simulink model "PasaBajo"  (R2020a)
settings: Solver=FixedStepAuto  StartTime=0.0  StopTime=6  FixedStep=0.003  RelTol=1e-3
undefined symbols (not defined in the file): wc
libraries: androidsensorlib x1
settings Model: Creator=luisi  LastModifiedBy=luisi
settings OptimizationCC: EnhancedBackFolding=on  PassReuseOutputArgsAs=Individual arguments  ZeroExternalMemoryAtStartup=off  ZeroInternalMemoryAtStartup=off  MaxStackSize=64  OptimizeBlockOrder=speed  DifferentSizesBufferReuse=on  EfficientTunableParamExpr=on
settings DebuggingCC: ParameterTunabilityLossMsg=error
settings HardwareCC: ProdBitPerPointer=32  ProdBitPerSizeT=32  ProdBitPerPtrDiffT=32  ProdLargestAtomicInteger=Long  ProdLargestAtomicFloat=Double  ProdWordSize=32  ProdHWDeviceType=ARM Compatible->ARM Cortex
settings SFSimCC: MATLABDynamicMemAlloc=off
settings RTWCC: SystemTargetFile=ert.tlc  HardwareBoard=Android Device  TemplateMakefile=ert_default_tmf  RTWVerbose=off  Toolchain=Android SDK/NDK Tools
settings CodeAppCC: ForceParamTrailComments=on  IgnoreCustomStorageClasses=off  OperatorAnnotations=on  SimulinkDataObjDesc=on  SFDataObjDesc=on  InsertBlockDesc=on
settings ERTTargetCC: SupportContinuousTime=on

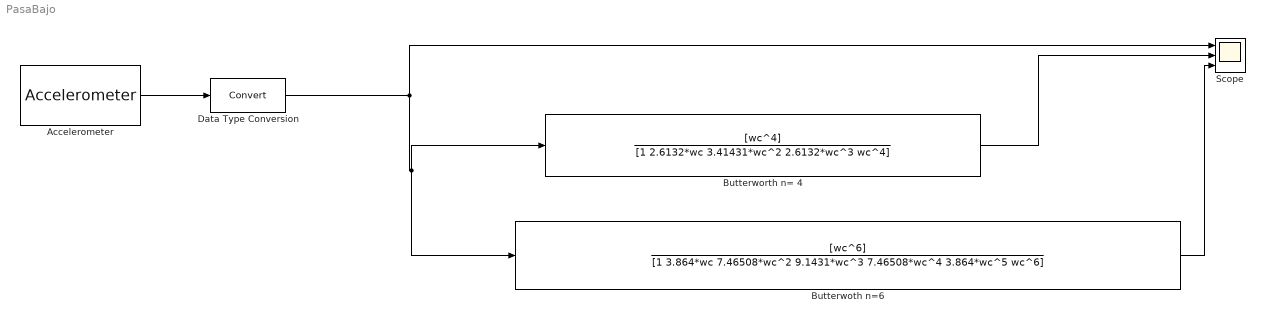
== system PasaBajo ==
  Accelerometer : androidsensorlib/Accelerometer  OutputVector=off  SampleTime=0.003  BlockPlatform=Android
      settings: SourceProductBaseCode=ANDROID
  Butterworth n= 4 : TransferFcn  Numerator=[wc^4]  Denominator=[1 2.6132*wc 3.41431*wc^2 2.6132*wc^3 wc^4]
  Butterwoth n=6 : TransferFcn  Numerator=[wc^6]  Denominator=[1 3.864*wc 7.46508*wc^2 9.1431*wc^3 7.46508*wc^4 3.864*wc^5 wc^6]
  Data Type Conversion : DataTypeConversion
  Scope : Scope  NumInputPorts=3
  wires:
  Data Type Conversion/1 -> Butterwoth n=6/1, Butterworth n= 4/1, Scope/1
  Accelerometer/2 -> Data Type Conversion/1
  Butterworth n= 4/1 -> Scope/2
  Butterwoth n=6/1 -> Scope/3
